simulink model "COSTEP_Exergy"  (R2024b)
settings: Solver=FixedStepAuto  StartTime=0.0  StopTime=25  FixedStep=1/3600  RelTol=1e-3
model workspace (MAT data in the model file):
  AD : Simulink.Parameter (value not decoded)
  AG : Simulink.Parameter (value not decoded)
  AH : Simulink.Parameter (value not decoded)
  AV : Simulink.Parameter (value not decoded)
  AVP : Simulink.Parameter (value not decoded)
  BCHL : Simulink.Parameter (value not decoded)
  BCHV : Simulink.Parameter (value not decoded)
  BD : Simulink.Parameter (value not decoded)
  BDIST : Simulink.Parameter (value not decoded)
  BG : Simulink.Parameter (value not decoded)
  BH : Simulink.Parameter (value not decoded)
  BVP : Simulink.Parameter (value not decoded)
  CD : Simulink.Parameter (value not decoded)
  CDIST : Simulink.Parameter (value not decoded)
  CG : Simulink.Parameter (value not decoded)
  CH : Simulink.Parameter (value not decoded)
  CVP : Simulink.Parameter (value not decoded)
  DDIST : Simulink.Parameter (value not decoded)
  DIST_CONST : Simulink.Parameter (value not decoded)
  ISV : Simulink.Parameter (value not decoded)
  TLAST : Simulink.Parameter (value not decoded)
  TNEXT : Simulink.Parameter (value not decoded)
  XMW : Simulink.Parameter (value not decoded)
  XNS : Simulink.Parameter (value not decoded)
  XNS2 : Simulink.Parameter (value not decoded)
  XNS3 : Simulink.Parameter (value not decoded)
  XNSADD : Simulink.Parameter (value not decoded)
  XNSE : Simulink.Parameter (value not decoded)
symbols that are objects in the model workspace (value not decoded): AD, AG, AH, AV, AVP, BD, BG, BH, BVP, CD, CG, CH, CVP, XMW, XNS, XNS2, XNS3, XNSE
undefined symbols (not defined in the file or in its folder): magnitude, msgbox, SETPT, XMEAS, XMV
libraries: mylib x403, dspindex x31
(part 11 of 13)

== system COSTEP_Exergy/Stream Measurements/Subsystem6/Separator recycle stream (after compressor)/Composition measurement mol%/Subsystem ==
  XST : Inport
  XMNSE : Inport  Port=2
  Bus Selector : BusSelector  OutputSignals=XMNSEA,XMNSEB,XMNSEC,XMNSED,XMNSEE,XMNSEF,XMNSEG,XMNSEH
  Process Noise I=23-{1..7,36} (8 alike) : mylib/Process Noise I=23-36  SystemSampleTime=-1  VariantActivationTime=update diagram  AllowFlexibleInterface=on  Latency=0  AutoFrameSizeCalculation=off
  Subsystem : Subsystem
  SMEASXA : Outport  VectorParamsAs1DForOutWhenUnconnected=off
  SMEASXB : Outport  Port=2  VectorParamsAs1DForOutWhenUnconnected=off
  SMEASXC : Outport  Port=3  VectorParamsAs1DForOutWhenUnconnected=off
  SMEASXD : Outport  Port=4  VectorParamsAs1DForOutWhenUnconnected=off
  SMEASXE : Outport  Port=5  VectorParamsAs1DForOutWhenUnconnected=off
  SMEASXF : Outport  Port=6  VectorParamsAs1DForOutWhenUnconnected=off
  SMEASXG : Outport  Port=7  VectorParamsAs1DForOutWhenUnconnected=off
  SMEASXH : Outport  Port=8  VectorParamsAs1DForOutWhenUnconnected=off
  wires:
  Process Noise I=23-36/1 -> SMEASXA/1
  Process Noise I=23-1/1 -> SMEASXB/1
  Bus Selector/2 -> Process Noise I=23-1/2  "<XMNSEB>"
  Process Noise I=23-2/1 -> SMEASXC/1
  Process Noise I=23-3/1 -> SMEASXD/1
  Process Noise I=23-4/1 -> SMEASXE/1
  Process Noise I=23-5/1 -> SMEASXF/1
  Process Noise I=23-6/1 -> SMEASXG/1
  Process Noise I=23-7/1 -> SMEASXH/1
  Bus Selector/7 -> Process Noise I=23-6/2  "<XMNSEG>"
  Bus Selector/8 -> Process Noise I=23-7/2  "<XMNSEH>"
  Bus Selector/6 -> Process Noise I=23-5/2  "<XMNSEF>"
  Bus Selector/5 -> Process Noise I=23-4/2  "<XMNSEE>"
  Bus Selector/4 -> Process Noise I=23-3/2  "<XMNSED>"
  Bus Selector/3 -> Process Noise I=23-2/2  "<XMNSEC>"
  Bus Selector/1 -> Process Noise I=23-36/2  "<XMNSEA>"
  XST/1 -> Subsystem/1(XST)
  Subsystem/1(XCMPA) -> Process Noise I=23-36/1
  Subsystem/2(XCMPB) -> Process Noise I=23-1/1
  Subsystem/3(XCMPC) -> Process Noise I=23-2/1
  Subsystem/4(XCMPD) -> Process Noise I=23-3/1
  Subsystem/5("XCMPE ") -> Process Noise I=23-4/1
  Subsystem/6("XCMPF ") -> Process Noise I=23-5/1
  Subsystem/7(XCMPG) -> Process Noise I=23-6/1
  Subsystem/8("XCMPH ") -> Process Noise I=23-7/1
  XMNSE/1 -> Bus Selector/1

== system COSTEP_Exergy/Stream Measurements/Subsystem6/Separator recycle stream (after compressor)/Flow measurement in kg//h/XMWS Molecular weight of Stream lb//lb-mol ==
  XST : Inport
  Product : Product
  Sum of Elements : Sum  Inputs=+
  "XMW(I) Molecular weight of components lb/lb-mol " : Constant  Value=XMW
  XMWS : Outport  VectorParamsAs1DForOutWhenUnconnected=off
  wires:
  Sum of Elements/1 -> XMWS/1
  Product/1 -> Sum of Elements/1
  XST/1 -> Product/1
  "XMW(I) Molecular weight of components lb/lb-mol "/1 -> Product/2

== system COSTEP_Exergy/Stream Measurements/Subsystem6/Separator recycle stream (after compressor)/Temperature measurement in C/TST(9) Temperature of Stream °C  ==
  HST : Inport  PortDimensions=1
  XLR : Inport  Port=2  PortDimensions=8
  ITY : Inport  Port=3
  "AG(I) Coefficient A to determine Enthalpy MBtu/lb·°F " : Constant  Value=AG
  "AH(I) Coefficient A to determine Enthalpy MBtu/lb·°F " : Constant  Value=AH
  AV(I) Coefficient AV to determine Enthalpy MBtu/lb : Constant  Value=AV
  BG(I) Coefficient B to determine Enthalpy MBtu/lb·°F² : Constant  Value=BG
  BH(I) Coefficient B to determine Enthalpy MBtu/lb·°F² : Constant  Value=BH
  CG(I) Coefficient C to determine Enthalpy MBtu/lb·°F³ : Constant  Value=CG
  CH(I) Coefficient C to determine Enthalpy MBtu/lb·°F³ : Constant  Value=CH
  Delay : Delay  DelayLength=1  InitialCondition=0
  MATLAB Function : MATLAB Function  TreatAsAtomicUnit=on
  "XMW(I) Molecular weight of components lb/lb-mol " : Constant  Value=XMW
  TST(9) : Outport  PortDimensions=1  VectorParamsAs1DForOutWhenUnconnected=off
  wires:
  MATLAB Function/1(TST) -> Delay/1, TST(9)/1
  Delay/1 -> MATLAB Function/12("TST ")
  "AG(I) Coefficient A to determine Enthalpy MBtu/lb·°F "/1 -> MATLAB Function/4(AG)
  AV(I) Coefficient AV to determine Enthalpy MBtu/lb/1 -> MATLAB Function/7(AV)
  HST/1 -> MATLAB Function/10(HST)
  CH(I) Coefficient C to determine Enthalpy MBtu/lb·°F³/1 -> MATLAB Function/3(CH)
  ITY/1 -> MATLAB Function/11(ITY)
  "XMW(I) Molecular weight of components lb/lb-mol "/1 -> MATLAB Function/8(XMW)
  XLR/1 -> MATLAB Function/9(XLR)
  "AH(I) Coefficient A to determine Enthalpy MBtu/lb·°F "/1 -> MATLAB Function/1(AH)
  CG(I) Coefficient C to determine Enthalpy MBtu/lb·°F³/1 -> MATLAB Function/6(CG)
  BH(I) Coefficient B to determine Enthalpy MBtu/lb·°F²/1 -> MATLAB Function/2(BH)
  BG(I) Coefficient B to determine Enthalpy MBtu/lb·°F²/1 -> MATLAB Function/5(BG)

== system COSTEP_Exergy/Stream Measurements/Subsystem6/Separator recycle stream (before compressor)/Composition measurement mol%/Subsystem ==
  XST : Inport
  XMNSE : Inport  Port=2
  Bus Selector : BusSelector  OutputSignals=XMNSEA,XMNSEB,XMNSEC,XMNSED,XMNSEE,XMNSEF,XMNSEG,XMNSEH
  Process Noise I=23-{1..7,36} (8 alike) : mylib/Process Noise I=23-36  SystemSampleTime=-1  VariantActivationTime=update diagram  AllowFlexibleInterface=on  Latency=0  AutoFrameSizeCalculation=off
  Subsystem : Subsystem
  SMEASXA : Outport  VectorParamsAs1DForOutWhenUnconnected=off
  SMEASXB : Outport  Port=2  VectorParamsAs1DForOutWhenUnconnected=off
  SMEASXC : Outport  Port=3  VectorParamsAs1DForOutWhenUnconnected=off
  SMEASXD : Outport  Port=4  VectorParamsAs1DForOutWhenUnconnected=off
  SMEASXE : Outport  Port=5  VectorParamsAs1DForOutWhenUnconnected=off
  SMEASXF : Outport  Port=6  VectorParamsAs1DForOutWhenUnconnected=off
  SMEASXG : Outport  Port=7  VectorParamsAs1DForOutWhenUnconnected=off
  SMEASXH : Outport  Port=8  VectorParamsAs1DForOutWhenUnconnected=off
  wires:
  Process Noise I=23-36/1 -> SMEASXA/1
  Process Noise I=23-1/1 -> SMEASXB/1
  Bus Selector/2 -> Process Noise I=23-1/2  "<XMNSEB>"
  Process Noise I=23-2/1 -> SMEASXC/1
  Process Noise I=23-3/1 -> SMEASXD/1
  Process Noise I=23-4/1 -> SMEASXE/1
  Process Noise I=23-5/1 -> SMEASXF/1
  Process Noise I=23-6/1 -> SMEASXG/1
  Process Noise I=23-7/1 -> SMEASXH/1
  Bus Selector/7 -> Process Noise I=23-6/2  "<XMNSEG>"
  Bus Selector/8 -> Process Noise I=23-7/2  "<XMNSEH>"
  Bus Selector/6 -> Process Noise I=23-5/2  "<XMNSEF>"
  Bus Selector/5 -> Process Noise I=23-4/2  "<XMNSEE>"
  Bus Selector/4 -> Process Noise I=23-3/2  "<XMNSED>"
  Bus Selector/3 -> Process Noise I=23-2/2  "<XMNSEC>"
  Bus Selector/1 -> Process Noise I=23-36/2  "<XMNSEA>"
  XST/1 -> Subsystem/1(XST)
  Subsystem/1(XCMPA) -> Process Noise I=23-36/1
  Subsystem/2(XCMPB) -> Process Noise I=23-1/1
  Subsystem/3(XCMPC) -> Process Noise I=23-2/1
  Subsystem/4(XCMPD) -> Process Noise I=23-3/1
  Subsystem/5("XCMPE ") -> Process Noise I=23-4/1
  Subsystem/6("XCMPF ") -> Process Noise I=23-5/1
  Subsystem/7(XCMPG) -> Process Noise I=23-6/1
  Subsystem/8("XCMPH ") -> Process Noise I=23-7/1
  XMNSE/1 -> Bus Selector/1

== system COSTEP_Exergy/Stream Measurements/Subsystem6/Separator recycle stream (before compressor)/Flow measurement in kg//h/XMWS Molecular weight of Stream lb//lb-mol ==
  XST : Inport
  Product : Product
  Sum of Elements : Sum  Inputs=+
  "XMW(I) Molecular weight of components lb/lb-mol " : Constant  Value=XMW
  XMWS : Outport  VectorParamsAs1DForOutWhenUnconnected=off
  wires:
  Sum of Elements/1 -> XMWS/1
  Product/1 -> Sum of Elements/1
  XST/1 -> Product/1
  "XMW(I) Molecular weight of components lb/lb-mol "/1 -> Product/2

== system COSTEP_Exergy/Stream Measurements/Subsystem6/Separator underflow stream/Composition measurement mol%/Subsystem ==
  XST : Inport
  XMNSE : Inport  Port=2
  Bus Selector : BusSelector  OutputSignals=XMNSED,XMNSEE,XMNSEF,XMNSEG,XMNSEH
  Process Noise I=23-{3..7} (5 alike) : mylib/Process Noise I=23-36  SystemSampleTime=-1  VariantActivationTime=update diagram  AllowFlexibleInterface=on  Latency=0  AutoFrameSizeCalculation=off
  Subsystem : Subsystem
  SMEASXD : Outport  VectorParamsAs1DForOutWhenUnconnected=off
  SMEASXE : Outport  Port=2  VectorParamsAs1DForOutWhenUnconnected=off
  SMEASXF : Outport  Port=3  VectorParamsAs1DForOutWhenUnconnected=off
  SMEASXG : Outport  Port=4  VectorParamsAs1DForOutWhenUnconnected=off
  SMEASXH : Outport  Port=5  VectorParamsAs1DForOutWhenUnconnected=off
  wires:
  Process Noise I=23-3/1 -> SMEASXD/1
  Process Noise I=23-4/1 -> SMEASXE/1
  Process Noise I=23-5/1 -> SMEASXF/1
  Process Noise I=23-6/1 -> SMEASXG/1
  Process Noise I=23-7/1 -> SMEASXH/1
  Bus Selector/4 -> Process Noise I=23-6/2  "<XMNSEG>"
  Bus Selector/5 -> Process Noise I=23-7/2  "<XMNSEH>"
  Bus Selector/3 -> Process Noise I=23-5/2  "<XMNSEF>"
  Bus Selector/2 -> Process Noise I=23-4/2  "<XMNSEE>"
  Bus Selector/1 -> Process Noise I=23-3/2  "<XMNSED>"
  XST/1 -> Subsystem/1(XST)
  Subsystem/1(XCMPD) -> Process Noise I=23-3/1
  Subsystem/2("XCMPE ") -> Process Noise I=23-4/1
  Subsystem/3("XCMPF ") -> Process Noise I=23-5/1
  Subsystem/4(XCMPG) -> Process Noise I=23-6/1
  Subsystem/5("XCMPH ") -> Process Noise I=23-7/1
  XMNSE/1 -> Bus Selector/1

== system COSTEP_Exergy/Stream Measurements/Subsystem6/Separator underflow stream/Flow measurement in kg//h/XMWS Molecular weight of Stream lb//lb-mol ==
  XST : Inport
  Product : Product
  Sum of Elements : Sum  Inputs=+
  "XMW(I) Molecular weight of components lb/lb-mol " : Constant  Value=XMW
  XMWS : Outport  VectorParamsAs1DForOutWhenUnconnected=off
  wires:
  Sum of Elements/1 -> XMWS/1
  Product/1 -> Sum of Elements/1
  XST/1 -> Product/1
  "XMW(I) Molecular weight of components lb/lb-mol "/1 -> Product/2

== system COSTEP_Exergy/Stream Measurements/Subsystem6/Stripper recycle stream/Composition measurement mol%/Subsystem ==
  XST : Inport
  XMNSE : Inport  Port=2
  Bus Selector : BusSelector  OutputSignals=XMNSEA,XMNSEB,XMNSEC,XMNSED,XMNSEE,XMNSEF,XMNSEG,XMNSEH
  Process Noise I=23-{1..7,36} (8 alike) : mylib/Process Noise I=23-36  SystemSampleTime=-1  VariantActivationTime=update diagram  AllowFlexibleInterface=on  Latency=0  AutoFrameSizeCalculation=off
  Subsystem : Subsystem
  SMEASXA : Outport  VectorParamsAs1DForOutWhenUnconnected=off
  SMEASXB : Outport  Port=2  VectorParamsAs1DForOutWhenUnconnected=off
  SMEASXC : Outport  Port=3  VectorParamsAs1DForOutWhenUnconnected=off
  SMEASXD : Outport  Port=4  VectorParamsAs1DForOutWhenUnconnected=off
  SMEASXE : Outport  Port=5  VectorParamsAs1DForOutWhenUnconnected=off
  SMEASXF : Outport  Port=6  VectorParamsAs1DForOutWhenUnconnected=off
  SMEASXG : Outport  Port=7  VectorParamsAs1DForOutWhenUnconnected=off
  SMEASXH : Outport  Port=8  VectorParamsAs1DForOutWhenUnconnected=off
  wires:
  Process Noise I=23-36/1 -> SMEASXA/1
  Process Noise I=23-1/1 -> SMEASXB/1
  Bus Selector/2 -> Process Noise I=23-1/2  "<XMNSEB>"
  Process Noise I=23-2/1 -> SMEASXC/1
  Process Noise I=23-3/1 -> SMEASXD/1
  Process Noise I=23-4/1 -> SMEASXE/1
  Process Noise I=23-5/1 -> SMEASXF/1
  Process Noise I=23-6/1 -> SMEASXG/1
  Process Noise I=23-7/1 -> SMEASXH/1
  Bus Selector/7 -> Process Noise I=23-6/2  "<XMNSEG>"
  Bus Selector/8 -> Process Noise I=23-7/2  "<XMNSEH>"
  Bus Selector/6 -> Process Noise I=23-5/2  "<XMNSEF>"
  Bus Selector/5 -> Process Noise I=23-4/2  "<XMNSEE>"
  Bus Selector/4 -> Process Noise I=23-3/2  "<XMNSED>"
  Bus Selector/3 -> Process Noise I=23-2/2  "<XMNSEC>"
  Bus Selector/1 -> Process Noise I=23-36/2  "<XMNSEA>"
  XST/1 -> Subsystem/1(XST)
  Subsystem/1(XCMPA) -> Process Noise I=23-36/1
  Subsystem/2(XCMPB) -> Process Noise I=23-1/1
  Subsystem/3(XCMPC) -> Process Noise I=23-2/1
  Subsystem/4(XCMPD) -> Process Noise I=23-3/1
  Subsystem/5("XCMPE ") -> Process Noise I=23-4/1
  Subsystem/6("XCMPF ") -> Process Noise I=23-5/1
  Subsystem/7(XCMPG) -> Process Noise I=23-6/1
  Subsystem/8("XCMPH ") -> Process Noise I=23-7/1
  XMNSE/1 -> Bus Selector/1

== system COSTEP_Exergy/Stream Measurements/Subsystem6/Stripper recycle stream/Flow measurement in kg//h/XMWS Molecular weight of Stream lb//lb-mol ==
  XST : Inport
  Product : Product
  Sum of Elements : Sum  Inputs=+
  "XMW(I) Molecular weight of components lb/lb-mol " : Constant  Value=XMW
  XMWS : Outport  VectorParamsAs1DForOutWhenUnconnected=off
  wires:
  Sum of Elements/1 -> XMWS/1
  Product/1 -> Sum of Elements/1
  XST/1 -> Product/1
  "XMW(I) Molecular weight of components lb/lb-mol "/1 -> Product/2

== system COSTEP_Exergy/Subsystem1/Condenser cooling water/CCin/Subsystem3/P Water Vapour Pressure Pa ==
  TK : Inport
  A Antoine Coefficient A : Constant  Value=11.6834
  Add : Sum
  Add1 : Sum  Inputs=+-
  B Antoine Coefficient B : Constant  Value=3816.44
  C Antoine Coefficient C : Constant  Value=-46.13
  Display1 : Display
  Divide : Product  Inputs=*/
  Divide1 : Product  Inputs=**
  Math Function : Math  SignedPower=on
  To Convert bar to Pa : Constant  Value=100000
  P : Outport  VectorParamsAs1DForOutWhenUnconnected=off
  wires:
  B Antoine Coefficient B/1 -> Divide/1
  C Antoine Coefficient C/1 -> Add/1
  A Antoine Coefficient A/1 -> Add1/1
  Add/1 -> Divide/2
  Divide/1 -> Add1/2
  Add1/1 -> Math Function/1
  TK/1 -> Add/2
  Math Function/1 -> Divide1/1
  Divide1/1 -> Display1/1, P/1
  To Convert bar to Pa/1 -> Divide1/2

== system COSTEP_Exergy/Subsystem1/Condenser cooling water/CCin/Subsystem3/Subsystem ==
  T1 : Inport
  T0 : Inport  Port=2
  Product3 : Product
  Subsystem2 : Subsystem
  Universal gas constant J/molK : Constant  Value=8.314
  h-h0 J/mol : Outport
  wires:
  T1/1 -> Subsystem2/1(T1)
  T0/1 -> Subsystem2/2(T0)
  Subsystem2/1(AT) -> Product3/1
  Universal gas constant J/molK/1 -> Product3/2
  Product3/1 -> h-h0 J/mol/1

== system COSTEP_Exergy/Subsystem1/Condenser cooling water/CCin/Subsystem3/Subsystem1 ==
  T1 : Inport
  T0 : Inport  Port=2
  P1 : Inport  Port=3
  P0 : Inport  Port=4
  " " : Product
  Add : Sum  Inputs=+-
  Display{1..8} (8 alike) : Display
  Divide : Product  Inputs=*/
  Math Function2 : Math  Operator=log  SignedPower=on
  Product3 : Product  Inputs=3
  Product6 : Product
  Subsystem : Subsystem
  Universal gas constant J/molK : Constant  Value=8.314
  T0(s-s0) J/mol : Outport
  wires:
  T1/1 -> Display6/1, Subsystem/1(T1)
  Subsystem/1(AT) -> Display8/1, Product3/1
  Universal gas constant J/molK/1 -> Product6/1, Product3/2
  T0/1 -> " "/1, Display7/1, Product3/3, Subsystem/2(T0)
  Math Function2/1 -> Display5/1, Product6/2
  Product6/1 -> Display4/1, " "/2
  Divide/1 -> Display2/1, Math Function2/1
  P0/1 -> Divide/2
  P1/1 -> Divide/1
  Product3/1 -> Add/1, Display3/1
  Add/1 -> T0(s-s0) J/mol/1
  " "/1 -> Add/2, Display1/1

== system COSTEP_Exergy/Subsystem1/Condenser cooling water/CCin/Subsystem3/Subsystem2 ==
  TC : Inport
  Temperature in Kelvin K : Sum
  To Convert °C to K : Constant  Value=273.15
  TK : Outport
  wires:
  TC/1 -> Temperature in Kelvin K/1
  Temperature in Kelvin K/1 -> TK/1
  To Convert °C to K/1 -> Temperature in Kelvin K/2

== system COSTEP_Exergy/Subsystem1/Condenser cooling water/CCout/Subsystem3/P Water Vapour Pressure Pa ==
  TK : Inport
  A Antoine Coefficient A : Constant  Value=11.6834
  Add : Sum
  Add1 : Sum  Inputs=+-
  B Antoine Coefficient B : Constant  Value=3816.44
  C Antoine Coefficient C : Constant  Value=-46.13
  Display1 : Display
  Divide : Product  Inputs=*/
  Divide1 : Product  Inputs=**
  Math Function : Math  SignedPower=on
  To Convert bar to Pa : Constant  Value=100000
  P : Outport  VectorParamsAs1DForOutWhenUnconnected=off
  wires:
  B Antoine Coefficient B/1 -> Divide/1
  C Antoine Coefficient C/1 -> Add/1
  A Antoine Coefficient A/1 -> Add1/1
  Add/1 -> Divide/2
  Divide/1 -> Add1/2
  Add1/1 -> Math Function/1
  TK/1 -> Add/2
  Math Function/1 -> Divide1/1
  Divide1/1 -> Display1/1, P/1
  To Convert bar to Pa/1 -> Divide1/2

== system COSTEP_Exergy/Subsystem1/Condenser cooling water/CCout/Subsystem3/Subsystem ==
  T1 : Inport
  T0 : Inport  Port=2
  Product3 : Product
  Subsystem2 : Subsystem
  Universal gas constant J/molK : Constant  Value=8.314
  h-h0 J/mol : Outport
  wires:
  T1/1 -> Subsystem2/1(T1)
  T0/1 -> Subsystem2/2(T0)
  Subsystem2/1(AT) -> Product3/1
  Universal gas constant J/molK/1 -> Product3/2
  Product3/1 -> h-h0 J/mol/1

== system COSTEP_Exergy/Subsystem1/Condenser cooling water/CCout/Subsystem3/Subsystem1 ==
  T1 : Inport
  T0 : Inport  Port=2
  P1 : Inport  Port=3
  P0 : Inport  Port=4
  " " : Product
  Add : Sum  Inputs=+-
  Display{1..8} (8 alike) : Display
  Divide : Product  Inputs=*/
  Math Function2 : Math  Operator=log  SignedPower=on
  Product3 : Product  Inputs=3
  Product6 : Product
  Subsystem : Subsystem
  Universal gas constant J/molK : Constant  Value=8.314
  T0(s-s0) J/mol : Outport
  wires:
  T1/1 -> Display6/1, Subsystem/1(T1)
  Subsystem/1(AT) -> Display8/1, Product3/1
  Universal gas constant J/molK/1 -> Product6/1, Product3/2
  T0/1 -> " "/1, Display7/1, Product3/3, Subsystem/2(T0)
  Math Function2/1 -> Display5/1, Product6/2
  Product6/1 -> Display4/1, " "/2
  Divide/1 -> Display2/1, Math Function2/1
  P0/1 -> Divide/2
  P1/1 -> Divide/1
  Product3/1 -> Add/1, Display3/1
  Add/1 -> T0(s-s0) J/mol/1
  " "/1 -> Add/2, Display1/1

== system COSTEP_Exergy/Subsystem1/Condenser cooling water/CCout/Subsystem3/Subsystem2 ==
  TC : Inport
  Temperature in Kelvin K : Sum
  To Convert °C to K : Constant  Value=273.15
  TK : Outport
  wires:
  TC/1 -> Temperature in Kelvin K/1
  Temperature in Kelvin K/1 -> TK/1
  To Convert °C to K/1 -> Temperature in Kelvin K/2

== system COSTEP_Exergy/Subsystem1/Reactor cooling water/RCin/Subsystem3/P Water Vapour Pressure Pa ==
  TK : Inport
  A Antoine Coefficient A : Constant  Value=11.6834
  Add : Sum
  Add1 : Sum  Inputs=+-
  B Antoine Coefficient B : Constant  Value=3816.44
  C Antoine Coefficient C : Constant  Value=-46.13
  Display1 : Display
  Divide : Product  Inputs=*/
  Divide1 : Product  Inputs=**
  Math Function : Math  SignedPower=on
  To Convert bar to Pa : Constant  Value=100000
  P : Outport  VectorParamsAs1DForOutWhenUnconnected=off
  wires:
  B Antoine Coefficient B/1 -> Divide/1
  C Antoine Coefficient C/1 -> Add/1
  A Antoine Coefficient A/1 -> Add1/1
  Add/1 -> Divide/2
  Divide/1 -> Add1/2
  Add1/1 -> Math Function/1
  TK/1 -> Add/2
  Math Function/1 -> Divide1/1
  Divide1/1 -> Display1/1, P/1
  To Convert bar to Pa/1 -> Divide1/2

== system COSTEP_Exergy/Subsystem1/Reactor cooling water/RCin/Subsystem3/Subsystem ==
  T1 : Inport
  T0 : Inport  Port=2
  Product3 : Product
  Subsystem2 : Subsystem
  Universal gas constant J/molK : Constant  Value=8.314
  h-h0 J/mol : Outport
  wires:
  T1/1 -> Subsystem2/1(T1)
  T0/1 -> Subsystem2/2(T0)
  Subsystem2/1(AT) -> Product3/1
  Universal gas constant J/molK/1 -> Product3/2
  Product3/1 -> h-h0 J/mol/1

== system COSTEP_Exergy/Subsystem1/Reactor cooling water/RCin/Subsystem3/Subsystem1 ==
  T1 : Inport
  T0 : Inport  Port=2
  P1 : Inport  Port=3
  P0 : Inport  Port=4
  " " : Product
  Add : Sum  Inputs=+-
  Display{1..8} (8 alike) : Display
  Divide : Product  Inputs=*/
  Math Function2 : Math  Operator=log  SignedPower=on
  Product3 : Product  Inputs=3
  Product6 : Product
  Subsystem : Subsystem
  Universal gas constant J/molK : Constant  Value=8.314
  T0(s-s0) J/mol : Outport
  wires:
  T1/1 -> Display6/1, Subsystem/1(T1)
  Subsystem/1(AT) -> Display8/1, Product3/1
  Universal gas constant J/molK/1 -> Product6/1, Product3/2
  T0/1 -> " "/1, Display7/1, Product3/3, Subsystem/2(T0)
  Math Function2/1 -> Display5/1, Product6/2
  Product6/1 -> Display4/1, " "/2
  Divide/1 -> Display2/1, Math Function2/1
  P0/1 -> Divide/2
  P1/1 -> Divide/1
  Product3/1 -> Add/1, Display3/1
  Add/1 -> T0(s-s0) J/mol/1
  " "/1 -> Add/2, Display1/1

== system COSTEP_Exergy/Subsystem1/Reactor cooling water/RCin/Subsystem3/Subsystem2 ==
  TC : Inport
  Temperature in Kelvin K : Sum
  To Convert °C to K : Constant  Value=273.15
  TK : Outport
  wires:
  TC/1 -> Temperature in Kelvin K/1
  Temperature in Kelvin K/1 -> TK/1
  To Convert °C to K/1 -> Temperature in Kelvin K/2

== system COSTEP_Exergy/Subsystem1/Reactor cooling water/RCout/Subsystem3/P Water Vapour Pressure Pa ==
  TK : Inport
  A Antoine Coefficient A : Constant  Value=11.6834
  Add : Sum
  Add1 : Sum  Inputs=+-
  B Antoine Coefficient B : Constant  Value=3816.44
  C Antoine Coefficient C : Constant  Value=-46.13
  Display1 : Display
  Divide : Product  Inputs=*/
  Divide1 : Product  Inputs=**
  Math Function : Math  SignedPower=on
  To Convert bar to Pa : Constant  Value=100000
  P : Outport  VectorParamsAs1DForOutWhenUnconnected=off
  wires:
  B Antoine Coefficient B/1 -> Divide/1
  C Antoine Coefficient C/1 -> Add/1
  A Antoine Coefficient A/1 -> Add1/1
  Add/1 -> Divide/2
  Divide/1 -> Add1/2
  Add1/1 -> Math Function/1
  TK/1 -> Add/2
  Math Function/1 -> Divide1/1
  Divide1/1 -> Display1/1, P/1
  To Convert bar to Pa/1 -> Divide1/2

== system COSTEP_Exergy/Subsystem1/Reactor cooling water/RCout/Subsystem3/Subsystem ==
  T1 : Inport
  T0 : Inport  Port=2
  Product3 : Product
  Subsystem2 : Subsystem
  Universal gas constant J/molK : Constant  Value=8.314
  h-h0 J/mol : Outport
  wires:
  T1/1 -> Subsystem2/1(T1)
  T0/1 -> Subsystem2/2(T0)
  Subsystem2/1(AT) -> Product3/1
  Universal gas constant J/molK/1 -> Product3/2
  Product3/1 -> h-h0 J/mol/1

== system COSTEP_Exergy/Subsystem1/Reactor cooling water/RCout/Subsystem3/Subsystem1 ==
  T1 : Inport
  T0 : Inport  Port=2
  P1 : Inport  Port=3
  P0 : Inport  Port=4
  " " : Product
  Add : Sum  Inputs=+-
  Display{1..8} (8 alike) : Display
  Divide : Product  Inputs=*/
  Math Function2 : Math  Operator=log  SignedPower=on
  Product3 : Product  Inputs=3
  Product6 : Product
  Subsystem : Subsystem
  Universal gas constant J/molK : Constant  Value=8.314
  T0(s-s0) J/mol : Outport
  wires:
  T1/1 -> Display6/1, Subsystem/1(T1)
  Subsystem/1(AT) -> Display8/1, Product3/1
  Universal gas constant J/molK/1 -> Product6/1, Product3/2
  T0/1 -> " "/1, Display7/1, Product3/3, Subsystem/2(T0)
  Math Function2/1 -> Display5/1, Product6/2
  Product6/1 -> Display4/1, " "/2
  Divide/1 -> Display2/1, Math Function2/1
  P0/1 -> Divide/2
  P1/1 -> Divide/1
  Product3/1 -> Add/1, Display3/1
  Add/1 -> T0(s-s0) J/mol/1
  " "/1 -> Add/2, Display1/1

== system COSTEP_Exergy/Subsystem1/Reactor cooling water/RCout/Subsystem3/Subsystem2 ==
  TC : Inport
  Temperature in Kelvin K : Sum
  To Convert °C to K : Constant  Value=273.15
  TK : Outport
  wires:
  TC/1 -> Temperature in Kelvin K/1
  Temperature in Kelvin K/1 -> TK/1
  To Convert °C to K/1 -> Temperature in Kelvin K/2

== system COSTEP_Exergy/Control Mode/Braatz/ /CONTROL 14/PI Control Setpoint Velocity form/Subsystem ==
  Setpoint : Inport
  Measurement : Inport  Port=2
  Controller Gain : Gain  Gain=Kc  SaturateOnIntegerOverflow=on  OutDataTypeStr=Inherit: Same as input  ParamDataTypeStr=Inherit: Same as input
  Error : ZeroOrderHold  SampleTime=Ts
  Error old : UnitDelay  SampleTime=Ts
  Gain : Gain  Gain=100/HS
  Gain1 : Gain  Gain=Ts/Ti  SaturateOnIntegerOverflow=on  OutDataTypeStr=Inherit: Same as input  ParamDataTypeStr=Inherit: Same as input
  Sum : Sum  Inputs=|+-  SaturateOnIntegerOverflow=on
  Sum1 : Sum  Inputs=++-  SaturateOnIntegerOverflow=on
  Delta Output : Outport
  wires:
  Measurement/1 -> Sum/2
  Controller Gain/1 -> Delta Output/1
  Gain1/1 -> Sum1/2
  Setpoint/1 -> Sum/1
  Error old/1 -> Sum1/3
  Sum1/1 -> Controller Gain/1
  Error/1 -> Sum1/1, Error old/1, Gain1/1
  Gain/1 -> Error/1
  Sum/1 -> Gain/1

== system COSTEP_Exergy/Control Mode/Braatz/ 10/CONTROL 6/P Control Velocity form/Pressure limits ==
  "XMV(6) " : Inport
  XMEAS : Inport  Port=2
  Abs : Abs  SaturateOnIntegerOverflow=off
  Bus Selector : BusSelector  OutputSignals=signal3.XMEAS(13)
  Constant : Constant  Value=100
  Constant1 : Constant  Value=0
  If : If  IfExpression=u1 >= 2950  ElseIfExpressions=u1 <= 2300
  If Action Subsystem : Subsystem  TreatAsAtomicUnit=on
  If Action Subsystem1 : Subsystem  TreatAsAtomicUnit=on
  If Action Subsystem2 : Subsystem  TreatAsAtomicUnit=on
  Merge : Merge  Inputs=3
  Valve Opening Limits : Saturate  UpperLimit=100  LowerLimit=0
  XMV(6) : Outport  VectorParamsAs1DForOutWhenUnconnected=off
  wires:
  If/1 -> If Action Subsystem/Action
  Constant1/1 -> If Action Subsystem1/1(In1)
  Merge/1 -> Abs/1
  If/3 -> If Action Subsystem2/Action
  Constant/1 -> If Action Subsystem/1(In1)
  Bus Selector/1 -> If/1  "<XMEAS(13)>"
  If Action Subsystem2/1(Out1) -> Merge/3
  If Action Subsystem1/1(Out1) -> Merge/2
  XMEAS/1 -> Bus Selector/1
  If/2 -> If Action Subsystem1/Action
  If Action Subsystem/1(Out1) -> Merge/1
  "XMV(6) "/1 -> If Action Subsystem2/1(In1)
  Abs/1 -> Valve Opening Limits/1
  Valve Opening Limits/1 -> XMV(6)/1

== system COSTEP_Exergy/Control Mode/Braatz/ 10/CONTROL 6/P Control Velocity form/Subsystem ==
  Setpoint : Inport
  Measurement : Inport  Port=2
  Controller Gain : Gain  Gain=Kc  SaturateOnIntegerOverflow=on  OutDataTypeStr=Inherit: Same as input  ParamDataTypeStr=Inherit: Same as input
  Error : ZeroOrderHold  SampleTime=Ts
  Error old : UnitDelay  SampleTime=Ts
  Gain : Gain  Gain=100/H
  Sum : Sum  Inputs=|+-  SaturateOnIntegerOverflow=on
  Sum1 : Sum  Inputs=+-  SaturateOnIntegerOverflow=on
  Delta Output : Outport
  wires:
  Gain/1 -> Error/1
  Sum/1 -> Gain/1
  Error/1 -> Error old/1, Sum1/1
  Sum1/1 -> Controller Gain/1
  Error old/1 -> Sum1/2
  Setpoint/1 -> Sum/1
  Controller Gain/1 -> Delta Output/1
  Measurement/1 -> Sum/2

== system COSTEP_Exergy/Random number generator/Stream Measurements SMEAS Gas analysis1/If Action Subsystem3/Subsystem/Stream 1/Subsystem ==
  G : Inport
  TESUB6 XMNSEA : Subsystem
  TESUB6 XMNSEB : Subsystem
  TESUB6 XMNSEC : Subsystem
  TESUB6 XMNSED : Subsystem
  TESUB6 XMNSEE : Subsystem
  TESUB6 XMNSEF : Subsystem
  TESUB6 XMNSEG : Subsystem
  TESUB6 XMNSEH : Subsystem
  XMNSEA : Outport  VectorParamsAs1DForOutWhenUnconnected=off
  XMNSEB : Outport  Port=2  VectorParamsAs1DForOutWhenUnconnected=off
  XMNSEC : Outport  Port=3  VectorParamsAs1DForOutWhenUnconnected=off
  XMNSED : Outport  Port=4  VectorParamsAs1DForOutWhenUnconnected=off
  XMNSEE : Outport  Port=5  VectorParamsAs1DForOutWhenUnconnected=off
  XMNSEF : Outport  Port=6  VectorParamsAs1DForOutWhenUnconnected=off
  XMNSEG : Outport  Port=7  VectorParamsAs1DForOutWhenUnconnected=off
  XMNSEH : Outport  Port=8  VectorParamsAs1DForOutWhenUnconnected=off
  G_NEW : Outport  Port=9  VectorParamsAs1DForOutWhenUnconnected=off
  wires:
  TESUB6 XMNSEB/2(G_NEW) -> TESUB6 XMNSEC/1(G)
  G/1 -> TESUB6 XMNSEA/1(G)
  TESUB6 XMNSEA/2(G_NEW) -> TESUB6 XMNSEB/1(G)
  TESUB6 XMNSEC/2(G_NEW) -> TESUB6 XMNSED/1(G)
  TESUB6 XMNSED/1(XMNSED) -> XMNSED/1  "XMNSED"
  TESUB6 XMNSEE/1(XMNSEE) -> XMNSEE/1  "XMNSEE"
  TESUB6 XMNSED/2(G_NEW) -> TESUB6 XMNSEE/1(G)
  TESUB6 XMNSEC/1(XMNSEC) -> XMNSEC/1  "XMNSEC"
  TESUB6 XMNSEA/1(XMNSEA) -> XMNSEA/1  "XMNSEA"
  TESUB6 XMNSEB/1(XMNSEB) -> XMNSEB/1  "XMNSEB"
  TESUB6 XMNSEE/2(G_NEW) -> TESUB6 XMNSEF/1(G)
  TESUB6 XMNSEF/2(G_NEW) -> TESUB6 XMNSEG/1(G)
  TESUB6 XMNSEG/2(G_NEW) -> TESUB6 XMNSEH/1(G)
  TESUB6 XMNSEH/2(G_NEW) -> G_NEW/1
  TESUB6 XMNSEF/1(XMNSEF) -> XMNSEF/1  "XMNSEF"
  TESUB6 XMNSEG/1(XMNSEG) -> XMNSEG/1  "XMNSEG"
  TESUB6 XMNSEH/1(XMNSEH) -> XMNSEH/1  "XMNSEH"

== system COSTEP_Exergy/Random number generator/Stream Measurements SMEAS Gas analysis1/If Action Subsystem3/Subsystem/Stream 13/Subsystem ==
  G : Inport
  TESUB6 XMNSEA : Subsystem
  TESUB6 XMNSEB : Subsystem
  TESUB6 XMNSEC : Subsystem
  TESUB6 XMNSED : Subsystem
  TESUB6 XMNSEE : Subsystem
  TESUB6 XMNSEF : Subsystem
  TESUB6 XMNSEG : Subsystem
  TESUB6 XMNSEH : Subsystem
  XMNSEA : Outport  VectorParamsAs1DForOutWhenUnconnected=off
  XMNSEB : Outport  Port=2  VectorParamsAs1DForOutWhenUnconnected=off
  XMNSEC : Outport  Port=3  VectorParamsAs1DForOutWhenUnconnected=off
  XMNSED : Outport  Port=4  VectorParamsAs1DForOutWhenUnconnected=off
  XMNSEE : Outport  Port=5  VectorParamsAs1DForOutWhenUnconnected=off
  XMNSEF : Outport  Port=6  VectorParamsAs1DForOutWhenUnconnected=off
  XMNSEG : Outport  Port=7  VectorParamsAs1DForOutWhenUnconnected=off
  XMNSEH : Outport  Port=8  VectorParamsAs1DForOutWhenUnconnected=off
  G_NEW : Outport  Port=9  VectorParamsAs1DForOutWhenUnconnected=off
  wires:
  TESUB6 XMNSEB/2(G_NEW) -> TESUB6 XMNSEC/1(G)
  G/1 -> TESUB6 XMNSEA/1(G)
  TESUB6 XMNSEA/2(G_NEW) -> TESUB6 XMNSEB/1(G)
  TESUB6 XMNSEC/2(G_NEW) -> TESUB6 XMNSED/1(G)
  TESUB6 XMNSED/1(XMNSED) -> XMNSED/1  "XMNSED"
  TESUB6 XMNSEE/1(XMNSEE) -> XMNSEE/1  "XMNSEE"
  TESUB6 XMNSED/2(G_NEW) -> TESUB6 XMNSEE/1(G)
  TESUB6 XMNSEC/1(XMNSEC) -> XMNSEC/1  "XMNSEC"
  TESUB6 XMNSEA/1(XMNSEA) -> XMNSEA/1  "XMNSEA"
  TESUB6 XMNSEB/1(XMNSEB) -> XMNSEB/1  "XMNSEB"
  TESUB6 XMNSEE/2(G_NEW) -> TESUB6 XMNSEF/1(G)
  TESUB6 XMNSEF/2(G_NEW) -> TESUB6 XMNSEG/1(G)
  TESUB6 XMNSEG/2(G_NEW) -> TESUB6 XMNSEH/1(G)
  TESUB6 XMNSEH/2(G_NEW) -> G_NEW/1
  TESUB6 XMNSEF/1(XMNSEF) -> XMNSEF/1  "XMNSEF"
  TESUB6 XMNSEG/1(XMNSEG) -> XMNSEG/1  "XMNSEG"
  TESUB6 XMNSEH/1(XMNSEH) -> XMNSEH/1  "XMNSEH"

== system COSTEP_Exergy/Random number generator/Stream Measurements SMEAS Gas analysis1/If Action Subsystem3/Subsystem/Stream 2/Subsystem ==
  G : Inport
  TESUB6 XMNSEA : Subsystem
  TESUB6 XMNSEB : Subsystem
  TESUB6 XMNSEC : Subsystem
  TESUB6 XMNSED : Subsystem
  TESUB6 XMNSEE : Subsystem
  TESUB6 XMNSEF : Subsystem
  TESUB6 XMNSEG : Subsystem
  TESUB6 XMNSEH : Subsystem
  XMNSEA : Outport  VectorParamsAs1DForOutWhenUnconnected=off
  XMNSEB : Outport  Port=2  VectorParamsAs1DForOutWhenUnconnected=off
  XMNSEC : Outport  Port=3  VectorParamsAs1DForOutWhenUnconnected=off
  XMNSED : Outport  Port=4  VectorParamsAs1DForOutWhenUnconnected=off
  XMNSEE : Outport  Port=5  VectorParamsAs1DForOutWhenUnconnected=off
  XMNSEF : Outport  Port=6  VectorParamsAs1DForOutWhenUnconnected=off
  XMNSEG : Outport  Port=7  VectorParamsAs1DForOutWhenUnconnected=off
  XMNSEH : Outport  Port=8  VectorParamsAs1DForOutWhenUnconnected=off
  G_NEW : Outport  Port=9  VectorParamsAs1DForOutWhenUnconnected=off
  wires:
  TESUB6 XMNSEB/2(G_NEW) -> TESUB6 XMNSEC/1(G)
  G/1 -> TESUB6 XMNSEA/1(G)
  TESUB6 XMNSEA/2(G_NEW) -> TESUB6 XMNSEB/1(G)
  TESUB6 XMNSEC/2(G_NEW) -> TESUB6 XMNSED/1(G)
  TESUB6 XMNSED/1(XMNSED) -> XMNSED/1  "XMNSED"
  TESUB6 XMNSEE/1(XMNSEE) -> XMNSEE/1  "XMNSEE"
  TESUB6 XMNSED/2(G_NEW) -> TESUB6 XMNSEE/1(G)
  TESUB6 XMNSEC/1(XMNSEC) -> XMNSEC/1  "XMNSEC"
  TESUB6 XMNSEA/1(XMNSEA) -> XMNSEA/1  "XMNSEA"
  TESUB6 XMNSEB/1(XMNSEB) -> XMNSEB/1  "XMNSEB"
  TESUB6 XMNSEE/2(G_NEW) -> TESUB6 XMNSEF/1(G)
  TESUB6 XMNSEF/2(G_NEW) -> TESUB6 XMNSEG/1(G)
  TESUB6 XMNSEG/2(G_NEW) -> TESUB6 XMNSEH/1(G)
  TESUB6 XMNSEH/2(G_NEW) -> G_NEW/1
  TESUB6 XMNSEF/1(XMNSEF) -> XMNSEF/1  "XMNSEF"
  TESUB6 XMNSEG/1(XMNSEG) -> XMNSEG/1  "XMNSEG"
  TESUB6 XMNSEH/1(XMNSEH) -> XMNSEH/1  "XMNSEH"

== system COSTEP_Exergy/Random number generator/Stream Measurements SMEAS Gas analysis1/If Action Subsystem3/Subsystem/Stream 3/Subsystem ==
  G : Inport
  TESUB6 XMNSEA : Subsystem
  TESUB6 XMNSEB : Subsystem
  TESUB6 XMNSEC : Subsystem
  TESUB6 XMNSED : Subsystem
  TESUB6 XMNSEE : Subsystem
  TESUB6 XMNSEF : Subsystem
  TESUB6 XMNSEG : Subsystem
  TESUB6 XMNSEH : Subsystem
  XMNSEA : Outport  VectorParamsAs1DForOutWhenUnconnected=off
  XMNSEB : Outport  Port=2  VectorParamsAs1DForOutWhenUnconnected=off
  XMNSEC : Outport  Port=3  VectorParamsAs1DForOutWhenUnconnected=off
  XMNSED : Outport  Port=4  VectorParamsAs1DForOutWhenUnconnected=off
  XMNSEE : Outport  Port=5  VectorParamsAs1DForOutWhenUnconnected=off
  XMNSEF : Outport  Port=6  VectorParamsAs1DForOutWhenUnconnected=off
  XMNSEG : Outport  Port=7  VectorParamsAs1DForOutWhenUnconnected=off
  XMNSEH : Outport  Port=8  VectorParamsAs1DForOutWhenUnconnected=off
  G_NEW : Outport  Port=9  VectorParamsAs1DForOutWhenUnconnected=off
  wires:
  TESUB6 XMNSEB/2(G_NEW) -> TESUB6 XMNSEC/1(G)
  G/1 -> TESUB6 XMNSEA/1(G)
  TESUB6 XMNSEA/2(G_NEW) -> TESUB6 XMNSEB/1(G)
  TESUB6 XMNSEC/2(G_NEW) -> TESUB6 XMNSED/1(G)
  TESUB6 XMNSED/1(XMNSED) -> XMNSED/1  "XMNSED"
  TESUB6 XMNSEE/1(XMNSEE) -> XMNSEE/1  "XMNSEE"
  TESUB6 XMNSED/2(G_NEW) -> TESUB6 XMNSEE/1(G)
  TESUB6 XMNSEC/1(XMNSEC) -> XMNSEC/1  "XMNSEC"
  TESUB6 XMNSEA/1(XMNSEA) -> XMNSEA/1  "XMNSEA"
  TESUB6 XMNSEB/1(XMNSEB) -> XMNSEB/1  "XMNSEB"
  TESUB6 XMNSEE/2(G_NEW) -> TESUB6 XMNSEF/1(G)
  TESUB6 XMNSEF/2(G_NEW) -> TESUB6 XMNSEG/1(G)
  TESUB6 XMNSEG/2(G_NEW) -> TESUB6 XMNSEH/1(G)
  TESUB6 XMNSEH/2(G_NEW) -> G_NEW/1
  TESUB6 XMNSEF/1(XMNSEF) -> XMNSEF/1  "XMNSEF"
  TESUB6 XMNSEG/1(XMNSEG) -> XMNSEG/1  "XMNSEG"
  TESUB6 XMNSEH/1(XMNSEH) -> XMNSEH/1  "XMNSEH"

== system COSTEP_Exergy/Random number generator/Stream Measurements SMEAS Gas analysis1/If Action Subsystem3/Subsystem/Stream 4/Subsystem ==
  G : Inport
  TESUB6 XMNSEA : Subsystem
  TESUB6 XMNSEB : Subsystem
  TESUB6 XMNSEC : Subsystem
  TESUB6 XMNSED : Subsystem
  TESUB6 XMNSEE : Subsystem
  TESUB6 XMNSEF : Subsystem
  TESUB6 XMNSEG : Subsystem
  TESUB6 XMNSEH : Subsystem
  XMNSEA : Outport  VectorParamsAs1DForOutWhenUnconnected=off
  XMNSEB : Outport  Port=2  VectorParamsAs1DForOutWhenUnconnected=off
  XMNSEC : Outport  Port=3  VectorParamsAs1DForOutWhenUnconnected=off
  XMNSED : Outport  Port=4  VectorParamsAs1DForOutWhenUnconnected=off
  XMNSEE : Outport  Port=5  VectorParamsAs1DForOutWhenUnconnected=off
  XMNSEF : Outport  Port=6  VectorParamsAs1DForOutWhenUnconnected=off
  XMNSEG : Outport  Port=7  VectorParamsAs1DForOutWhenUnconnected=off
  XMNSEH : Outport  Port=8  VectorParamsAs1DForOutWhenUnconnected=off
  G_NEW : Outport  Port=9  VectorParamsAs1DForOutWhenUnconnected=off
  wires:
  TESUB6 XMNSEB/2(G_NEW) -> TESUB6 XMNSEC/1(G)
  G/1 -> TESUB6 XMNSEA/1(G)
  TESUB6 XMNSEA/2(G_NEW) -> TESUB6 XMNSEB/1(G)
  TESUB6 XMNSEC/2(G_NEW) -> TESUB6 XMNSED/1(G)
  TESUB6 XMNSED/1(XMNSED) -> XMNSED/1  "XMNSED"
  TESUB6 XMNSEE/1(XMNSEE) -> XMNSEE/1  "XMNSEE"
  TESUB6 XMNSED/2(G_NEW) -> TESUB6 XMNSEE/1(G)
  TESUB6 XMNSEC/1(XMNSEC) -> XMNSEC/1  "XMNSEC"
  TESUB6 XMNSEA/1(XMNSEA) -> XMNSEA/1  "XMNSEA"
  TESUB6 XMNSEB/1(XMNSEB) -> XMNSEB/1  "XMNSEB"
  TESUB6 XMNSEE/2(G_NEW) -> TESUB6 XMNSEF/1(G)
  TESUB6 XMNSEF/2(G_NEW) -> TESUB6 XMNSEG/1(G)
  TESUB6 XMNSEG/2(G_NEW) -> TESUB6 XMNSEH/1(G)
  TESUB6 XMNSEH/2(G_NEW) -> G_NEW/1
  TESUB6 XMNSEF/1(XMNSEF) -> XMNSEF/1  "XMNSEF"
  TESUB6 XMNSEG/1(XMNSEG) -> XMNSEG/1  "XMNSEG"
  TESUB6 XMNSEH/1(XMNSEH) -> XMNSEH/1  "XMNSEH"

== system COSTEP_Exergy/Random number generator/Stream Measurements SMEAS Gas analysis1/If Action Subsystem3/Subsystem/Stream 5/Subsystem ==
  G : Inport
  TESUB6 XMNSEA : Subsystem
  TESUB6 XMNSEB : Subsystem
  TESUB6 XMNSEC : Subsystem
  TESUB6 XMNSED : Subsystem
  TESUB6 XMNSEE : Subsystem
  TESUB6 XMNSEF : Subsystem
  TESUB6 XMNSEG : Subsystem
  TESUB6 XMNSEH : Subsystem
  XMNSEA : Outport  VectorParamsAs1DForOutWhenUnconnected=off
  XMNSEB : Outport  Port=2  VectorParamsAs1DForOutWhenUnconnected=off
  XMNSEC : Outport  Port=3  VectorParamsAs1DForOutWhenUnconnected=off
  XMNSED : Outport  Port=4  VectorParamsAs1DForOutWhenUnconnected=off
  XMNSEE : Outport  Port=5  VectorParamsAs1DForOutWhenUnconnected=off
  XMNSEF : Outport  Port=6  VectorParamsAs1DForOutWhenUnconnected=off
  XMNSEG : Outport  Port=7  VectorParamsAs1DForOutWhenUnconnected=off
  XMNSEH : Outport  Port=8  VectorParamsAs1DForOutWhenUnconnected=off
  G_NEW : Outport  Port=9  VectorParamsAs1DForOutWhenUnconnected=off
  wires:
  TESUB6 XMNSEB/2(G_NEW) -> TESUB6 XMNSEC/1(G)
  G/1 -> TESUB6 XMNSEA/1(G)
  TESUB6 XMNSEA/2(G_NEW) -> TESUB6 XMNSEB/1(G)
  TESUB6 XMNSEC/2(G_NEW) -> TESUB6 XMNSED/1(G)
  TESUB6 XMNSED/1(XMNSED) -> XMNSED/1  "XMNSED"
  TESUB6 XMNSEE/1(XMNSEE) -> XMNSEE/1  "XMNSEE"
  TESUB6 XMNSED/2(G_NEW) -> TESUB6 XMNSEE/1(G)
  TESUB6 XMNSEC/1(XMNSEC) -> XMNSEC/1  "XMNSEC"
  TESUB6 XMNSEA/1(XMNSEA) -> XMNSEA/1  "XMNSEA"
  TESUB6 XMNSEB/1(XMNSEB) -> XMNSEB/1  "XMNSEB"
  TESUB6 XMNSEE/2(G_NEW) -> TESUB6 XMNSEF/1(G)
  TESUB6 XMNSEF/2(G_NEW) -> TESUB6 XMNSEG/1(G)
  TESUB6 XMNSEG/2(G_NEW) -> TESUB6 XMNSEH/1(G)
  TESUB6 XMNSEH/2(G_NEW) -> G_NEW/1
  TESUB6 XMNSEF/1(XMNSEF) -> XMNSEF/1  "XMNSEF"
  TESUB6 XMNSEG/1(XMNSEG) -> XMNSEG/1  "XMNSEG"
  TESUB6 XMNSEH/1(XMNSEH) -> XMNSEH/1  "XMNSEH"

== system COSTEP_Exergy/Random number generator/Stream Measurements SMEAS Gas analysis1/If Action Subsystem3/Subsystem/Stream 6/Subsystem ==
  G : Inport
  TESUB6 XMNSEA : Subsystem
  TESUB6 XMNSEB : Subsystem
  TESUB6 XMNSEC : Subsystem
  TESUB6 XMNSED : Subsystem
  TESUB6 XMNSEE : Subsystem
  TESUB6 XMNSEF : Subsystem
  TESUB6 XMNSEG : Subsystem
  TESUB6 XMNSEH : Subsystem
  XMNSEA : Outport  VectorParamsAs1DForOutWhenUnconnected=off
  XMNSEB : Outport  Port=2  VectorParamsAs1DForOutWhenUnconnected=off
  XMNSEC : Outport  Port=3  VectorParamsAs1DForOutWhenUnconnected=off
  XMNSED : Outport  Port=4  VectorParamsAs1DForOutWhenUnconnected=off
  XMNSEE : Outport  Port=5  VectorParamsAs1DForOutWhenUnconnected=off
  XMNSEF : Outport  Port=6  VectorParamsAs1DForOutWhenUnconnected=off
  XMNSEG : Outport  Port=7  VectorParamsAs1DForOutWhenUnconnected=off
  XMNSEH : Outport  Port=8  VectorParamsAs1DForOutWhenUnconnected=off
  G_NEW : Outport  Port=9  VectorParamsAs1DForOutWhenUnconnected=off
  wires:
  TESUB6 XMNSEB/2(G_NEW) -> TESUB6 XMNSEC/1(G)
  G/1 -> TESUB6 XMNSEA/1(G)
  TESUB6 XMNSEA/2(G_NEW) -> TESUB6 XMNSEB/1(G)
  TESUB6 XMNSEC/2(G_NEW) -> TESUB6 XMNSED/1(G)
  TESUB6 XMNSED/1(XMNSED) -> XMNSED/1  "XMNSED"
  TESUB6 XMNSEE/1(XMNSEE) -> XMNSEE/1  "XMNSEE"
  TESUB6 XMNSED/2(G_NEW) -> TESUB6 XMNSEE/1(G)
  TESUB6 XMNSEC/1(XMNSEC) -> XMNSEC/1  "XMNSEC"
  TESUB6 XMNSEA/1(XMNSEA) -> XMNSEA/1  "XMNSEA"
  TESUB6 XMNSEB/1(XMNSEB) -> XMNSEB/1  "XMNSEB"
  TESUB6 XMNSEE/2(G_NEW) -> TESUB6 XMNSEF/1(G)
  TESUB6 XMNSEF/2(G_NEW) -> TESUB6 XMNSEG/1(G)
  TESUB6 XMNSEG/2(G_NEW) -> TESUB6 XMNSEH/1(G)
  TESUB6 XMNSEH/2(G_NEW) -> G_NEW/1
  TESUB6 XMNSEF/1(XMNSEF) -> XMNSEF/1  "XMNSEF"
  TESUB6 XMNSEG/1(XMNSEG) -> XMNSEG/1  "XMNSEG"
  TESUB6 XMNSEH/1(XMNSEH) -> XMNSEH/1  "XMNSEH"

== system COSTEP_Exergy/Random number generator/Stream Measurements SMEAS Gas analysis1/If Action Subsystem3/Subsystem/Stream 8/Subsystem ==
  G : Inport
  TESUB6 XMNSEA : Subsystem
  TESUB6 XMNSEB : Subsystem
  TESUB6 XMNSEC : Subsystem
  TESUB6 XMNSED : Subsystem
  TESUB6 XMNSEE : Subsystem
  TESUB6 XMNSEF : Subsystem
  TESUB6 XMNSEG : Subsystem
  TESUB6 XMNSEH : Subsystem
  XMNSEA : Outport  VectorParamsAs1DForOutWhenUnconnected=off
  XMNSEB : Outport  Port=2  VectorParamsAs1DForOutWhenUnconnected=off
  XMNSEC : Outport  Port=3  VectorParamsAs1DForOutWhenUnconnected=off
  XMNSED : Outport  Port=4  VectorParamsAs1DForOutWhenUnconnected=off
  XMNSEE : Outport  Port=5  VectorParamsAs1DForOutWhenUnconnected=off
  XMNSEF : Outport  Port=6  VectorParamsAs1DForOutWhenUnconnected=off
  XMNSEG : Outport  Port=7  VectorParamsAs1DForOutWhenUnconnected=off
  XMNSEH : Outport  Port=8  VectorParamsAs1DForOutWhenUnconnected=off
  G_NEW : Outport  Port=9  VectorParamsAs1DForOutWhenUnconnected=off
  wires:
  TESUB6 XMNSEB/2(G_NEW) -> TESUB6 XMNSEC/1(G)
  G/1 -> TESUB6 XMNSEA/1(G)
  TESUB6 XMNSEA/2(G_NEW) -> TESUB6 XMNSEB/1(G)
  TESUB6 XMNSEC/2(G_NEW) -> TESUB6 XMNSED/1(G)
  TESUB6 XMNSED/1(XMNSED) -> XMNSED/1  "XMNSED"
  TESUB6 XMNSEE/1(XMNSEE) -> XMNSEE/1  "XMNSEE"
  TESUB6 XMNSED/2(G_NEW) -> TESUB6 XMNSEE/1(G)
  TESUB6 XMNSEC/1(XMNSEC) -> XMNSEC/1  "XMNSEC"
  TESUB6 XMNSEA/1(XMNSEA) -> XMNSEA/1  "XMNSEA"
  TESUB6 XMNSEB/1(XMNSEB) -> XMNSEB/1  "XMNSEB"
  TESUB6 XMNSEE/2(G_NEW) -> TESUB6 XMNSEF/1(G)
  TESUB6 XMNSEF/2(G_NEW) -> TESUB6 XMNSEG/1(G)
  TESUB6 XMNSEG/2(G_NEW) -> TESUB6 XMNSEH/1(G)
  TESUB6 XMNSEH/2(G_NEW) -> G_NEW/1
  TESUB6 XMNSEF/1(XMNSEF) -> XMNSEF/1  "XMNSEF"
  TESUB6 XMNSEG/1(XMNSEG) -> XMNSEG/1  "XMNSEG"
  TESUB6 XMNSEH/1(XMNSEH) -> XMNSEH/1  "XMNSEH"

== system COSTEP_Exergy/Random number generator/Stream Measurements SMEAS Gas analysis1/If Action Subsystem3/Subsystem/Stream 9/Subsystem ==
  G : Inport
  TESUB6 XMNSEA : Subsystem
  TESUB6 XMNSEB : Subsystem
  TESUB6 XMNSEC : Subsystem
  TESUB6 XMNSED : Subsystem
  TESUB6 XMNSEE : Subsystem
  TESUB6 XMNSEF : Subsystem
  TESUB6 XMNSEG : Subsystem
  TESUB6 XMNSEH : Subsystem
  XMNSEA : Outport  VectorParamsAs1DForOutWhenUnconnected=off
  XMNSEB : Outport  Port=2  VectorParamsAs1DForOutWhenUnconnected=off
  XMNSEC : Outport  Port=3  VectorParamsAs1DForOutWhenUnconnected=off
  XMNSED : Outport  Port=4  VectorParamsAs1DForOutWhenUnconnected=off
  XMNSEE : Outport  Port=5  VectorParamsAs1DForOutWhenUnconnected=off
  XMNSEF : Outport  Port=6  VectorParamsAs1DForOutWhenUnconnected=off
  XMNSEG : Outport  Port=7  VectorParamsAs1DForOutWhenUnconnected=off
  XMNSEH : Outport  Port=8  VectorParamsAs1DForOutWhenUnconnected=off
  G_NEW : Outport  Port=9  VectorParamsAs1DForOutWhenUnconnected=off
  wires:
  TESUB6 XMNSEB/2(G_NEW) -> TESUB6 XMNSEC/1(G)
  G/1 -> TESUB6 XMNSEA/1(G)
  TESUB6 XMNSEA/2(G_NEW) -> TESUB6 XMNSEB/1(G)
  TESUB6 XMNSEC/2(G_NEW) -> TESUB6 XMNSED/1(G)
  TESUB6 XMNSED/1(XMNSED) -> XMNSED/1  "XMNSED"
  TESUB6 XMNSEE/1(XMNSEE) -> XMNSEE/1  "XMNSEE"
  TESUB6 XMNSED/2(G_NEW) -> TESUB6 XMNSEE/1(G)
  TESUB6 XMNSEC/1(XMNSEC) -> XMNSEC/1  "XMNSEC"
  TESUB6 XMNSEA/1(XMNSEA) -> XMNSEA/1  "XMNSEA"
  TESUB6 XMNSEB/1(XMNSEB) -> XMNSEB/1  "XMNSEB"
  TESUB6 XMNSEE/2(G_NEW) -> TESUB6 XMNSEF/1(G)
  TESUB6 XMNSEF/2(G_NEW) -> TESUB6 XMNSEG/1(G)
  TESUB6 XMNSEG/2(G_NEW) -> TESUB6 XMNSEH/1(G)
  TESUB6 XMNSEH/2(G_NEW) -> G_NEW/1
  TESUB6 XMNSEF/1(XMNSEF) -> XMNSEF/1  "XMNSEF"
  TESUB6 XMNSEG/1(XMNSEG) -> XMNSEG/1  "XMNSEG"
  TESUB6 XMNSEH/1(XMNSEH) -> XMNSEH/1  "XMNSEH"

== system COSTEP_Exergy/Random number generator/Stream Measurements SMEAS Product analysis1/If Action Subsystem3/Subsystem/Subsystem1/Subsystem ==
  G : Inport
  TESUB6 XMNSED : Subsystem
  TESUB6 XMNSEE : Subsystem
  TESUB6 XMNSEF : Subsystem
  TESUB6 XMNSEG : Subsystem
  TESUB6 XMNSEH : Subsystem
  XMNSED : Outport  VectorParamsAs1DForOutWhenUnconnected=off
  XMNSEE : Outport  Port=2  VectorParamsAs1DForOutWhenUnconnected=off
  XMNSEF : Outport  Port=3  VectorParamsAs1DForOutWhenUnconnected=off
  XMNSEG : Outport  Port=4  VectorParamsAs1DForOutWhenUnconnected=off
  XMNSEH : Outport  Port=5  VectorParamsAs1DForOutWhenUnconnected=off
  G_NEW : Outport  Port=6  VectorParamsAs1DForOutWhenUnconnected=off
  wires:
  TESUB6 XMNSEE/2(G_NEW) -> TESUB6 XMNSEF/1(G)
  G/1 -> TESUB6 XMNSED/1(G)
  TESUB6 XMNSED/2(G_NEW) -> TESUB6 XMNSEE/1(G)
  TESUB6 XMNSEF/2(G_NEW) -> TESUB6 XMNSEG/1(G)
  TESUB6 XMNSEG/1(XMNS) -> XMNSEG/1  "XMNSEG"
  TESUB6 XMNSEH/1(XMNS) -> XMNSEH/1  "XMNSEH"
  TESUB6 XMNSEH/2(G_NEW) -> G_NEW/1
  TESUB6 XMNSEG/2(G_NEW) -> TESUB6 XMNSEH/1(G)
  TESUB6 XMNSEF/1(XMNS) -> XMNSEF/1  "XMNSEF"
  TESUB6 XMNSED/1(XMNS) -> XMNSED/1  "XMNSED"
  TESUB6 XMNSEE/1(XMNS) -> XMNSEE/1  "XMNSEE"

== system COSTEP_Exergy/Random number generator/Stream Measurements SMEAS Product analysis1/If Action Subsystem3/Subsystem/Subsystem2/Subsystem ==
  G : Inport
  TESUB6 XMNSED : Subsystem
  TESUB6 XMNSEE : Subsystem
  TESUB6 XMNSEF : Subsystem
  TESUB6 XMNSEG : Subsystem
  TESUB6 XMNSEH : Subsystem
  XMNSED : Outport  VectorParamsAs1DForOutWhenUnconnected=off
  XMNSEE : Outport  Port=2  VectorParamsAs1DForOutWhenUnconnected=off
  XMNSEF : Outport  Port=3  VectorParamsAs1DForOutWhenUnconnected=off
  XMNSEG : Outport  Port=4  VectorParamsAs1DForOutWhenUnconnected=off
  XMNSEH : Outport  Port=5  VectorParamsAs1DForOutWhenUnconnected=off
  G_NEW : Outport  Port=6  VectorParamsAs1DForOutWhenUnconnected=off
  wires:
  TESUB6 XMNSEE/2(G_NEW) -> TESUB6 XMNSEF/1(G)
  G/1 -> TESUB6 XMNSED/1(G)
  TESUB6 XMNSED/2(G_NEW) -> TESUB6 XMNSEE/1(G)
  TESUB6 XMNSEF/2(G_NEW) -> TESUB6 XMNSEG/1(G)
  TESUB6 XMNSEG/1(XMNS) -> XMNSEG/1  "XMNSEG"
  TESUB6 XMNSEH/1(XMNS) -> XMNSEH/1  "XMNSEH"
  TESUB6 XMNSEH/2(G_NEW) -> G_NEW/1
  TESUB6 XMNSEG/2(G_NEW) -> TESUB6 XMNSEH/1(G)
  TESUB6 XMNSEF/1(XMNS) -> XMNSEF/1  "XMNSEF"
  TESUB6 XMNSED/1(XMNS) -> XMNSED/1  "XMNSED"
  TESUB6 XMNSEE/1(XMNS) -> XMNSEE/1  "XMNSEE"

== system COSTEP_Exergy/Stream Measurements/Subsystem6/A and C feed stream/Composition measurement mol%/Subsystem/Subsystem ==
  XST : Inport
  Constant : Constant  Value=100
  Multiport Selector : dspindex/Multiport Selector  rowsOrCols=Rows  idxCellArray={ 1,2,3}  idxErrMode=Clip Index
  Product : Product
  Product1 : Product
  Product2 : Product
  XCMPA : Outport  VectorParamsAs1DForOutWhenUnconnected=off
  XCMPB : Outport  Port=2  VectorParamsAs1DForOutWhenUnconnected=off
  XCMPC : Outport  Port=3  VectorParamsAs1DForOutWhenUnconnected=off
  wires:
  Multiport Selector/1 -> Product/1
  Multiport Selector/3 -> Product2/1
  Constant/1 -> Product/2, Product1/2, Product2/2
  XST/1 -> Multiport Selector/1
  Multiport Selector/2 -> Product1/1
  Product/1 -> XCMPA/1
  Product1/1 -> XCMPB/1
  Product2/1 -> XCMPC/1

== system COSTEP_Exergy/Stream Measurements/Subsystem6/A feed stream/Composition measurement mol%/Subsystem/Subsystem ==
  XST : Inport
  Constant : Constant  Value=100
  Multiport Selector : dspindex/Multiport Selector  rowsOrCols=Rows  idxCellArray={ 1,2}  idxErrMode=Clip Index
  Product : Product
  Product1 : Product
  XCMPA : Outport  VectorParamsAs1DForOutWhenUnconnected=off
  XCMPB : Outport  Port=2  VectorParamsAs1DForOutWhenUnconnected=off
  wires:
  Multiport Selector/1 -> Product/1
  Constant/1 -> Product/2, Product1/2
  XST/1 -> Multiport Selector/1
  Multiport Selector/2 -> Product1/1
  Product/1 -> XCMPA/1
  Product1/1 -> XCMPB/1

== system COSTEP_Exergy/Stream Measurements/Subsystem6/Condenser product stream/Composition measurement mol%/Subsystem/Subsystem ==
  XST : Inport
  Constant : Constant  Value=100
  Multiport Selector : dspindex/Multiport Selector  rowsOrCols=Rows  idxCellArray={ 1,2,3,4,5,6,7,8}  idxErrMode=Clip Index
  Product{,1..7} (8 alike) : Product
  XCMPA : Outport  VectorParamsAs1DForOutWhenUnconnected=off
  XCMPB : Outport  Port=2  VectorParamsAs1DForOutWhenUnconnected=off
  XCMPC : Outport  Port=3  VectorParamsAs1DForOutWhenUnconnected=off
  XCMPD : Outport  Port=4  VectorParamsAs1DForOutWhenUnconnected=off
  "XCMPE " : Outport  Port=5  VectorParamsAs1DForOutWhenUnconnected=off
  "XCMPF " : Outport  Port=6  VectorParamsAs1DForOutWhenUnconnected=off
  XCMPG : Outport  Port=7  VectorParamsAs1DForOutWhenUnconnected=off
  "XCMPH " : Outport  Port=8  VectorParamsAs1DForOutWhenUnconnected=off
  wires:
  Multiport Selector/6 -> Product5/1
  Multiport Selector/8 -> Product7/1
  Multiport Selector/5 -> Product4/1
  Multiport Selector/7 -> Product6/1
  Multiport Selector/1 -> Product/1
  Multiport Selector/3 -> Product2/1
  Constant/1 -> Product/2, Product1/2, Product2/2, Product3/2, Product4/2, Product5/2, Product7/2, Product6/2
  Multiport Selector/4 -> Product3/1
  XST/1 -> Multiport Selector/1
  Multiport Selector/2 -> Product1/1
  Product/1 -> XCMPA/1
  Product1/1 -> XCMPB/1
  Product2/1 -> XCMPC/1
  Product3/1 -> XCMPD/1
  Product4/1 -> "XCMPE "/1
  Product5/1 -> "XCMPF "/1
  Product6/1 -> XCMPG/1
  Product7/1 -> "XCMPH "/1

== system COSTEP_Exergy/Stream Measurements/Subsystem6/D feed stream/Composition measurement mol%/Subsystem/Subsystem ==
  XST : Inport
  Constant : Constant  Value=100
  Multiport Selector : dspindex/Multiport Selector  rowsOrCols=Rows  idxCellArray={ 2,4}  idxErrMode=Clip Index
  Product : Product
  Product1 : Product
  XCMPB : Outport  VectorParamsAs1DForOutWhenUnconnected=off
  XCMPD : Outport  Port=2  VectorParamsAs1DForOutWhenUnconnected=off
  wires:
  Multiport Selector/1 -> Product/1
  Constant/1 -> Product/2, Product1/2
  XST/1 -> Multiport Selector/1
  Multiport Selector/2 -> Product1/1
  Product/1 -> XCMPB/1
  Product1/1 -> XCMPD/1
